simulink model "PID"  (R2017a)
settings: Solver=ode45  StartTime=0.0  StopTime=10.0  RelTol=1e-3  EnableMultiTasking=on
libraries: powerlib_meascontrol x3, simulink x1
settings Model: Creator=fangtiqiang  LastModifiedBy=fangtiqiang
settings DataIOCC: LimitDataPoints=on  SaveFormat=Array
settings OptimizationCC: LifeSpan=inf
settings DebuggingCC: SolverPrmCheckMsg=warning  SFUnexpectedBacktrackingDiag=warning  SFNoUnconditionalDefaultTransitionDiag=warning  SFExecutionAtInitializationDiag=none
settings HardwareCC: ProdBitPerPointer=32  ProdBitPerSizeT=32  ProdBitPerPtrDiffT=32  ProdLargestAtomicFloat=None  ProdIntDivRoundTo=Undefined  ProdEndianess=Unspecified  ProdWordSize=32  ProdHWDeviceType=32-bit Generic
settings ModelReferenceCC: PropagateSignalLabelsOutOfModel=off
settings GRTTargetCC: TargetLangStandard=C89/C90 (ANSI)  GeneratePreprocessorConditionals=Disable all
settings ConfigComp: CovMetricSettings=dw  CovHtmlReporting=on  CovSaveCumulativeToWorkspaceVar=on  CovSaveSingleToWorkspaceVar=on  CovExternalEMLEnable=off  CovSFcnEnable=off

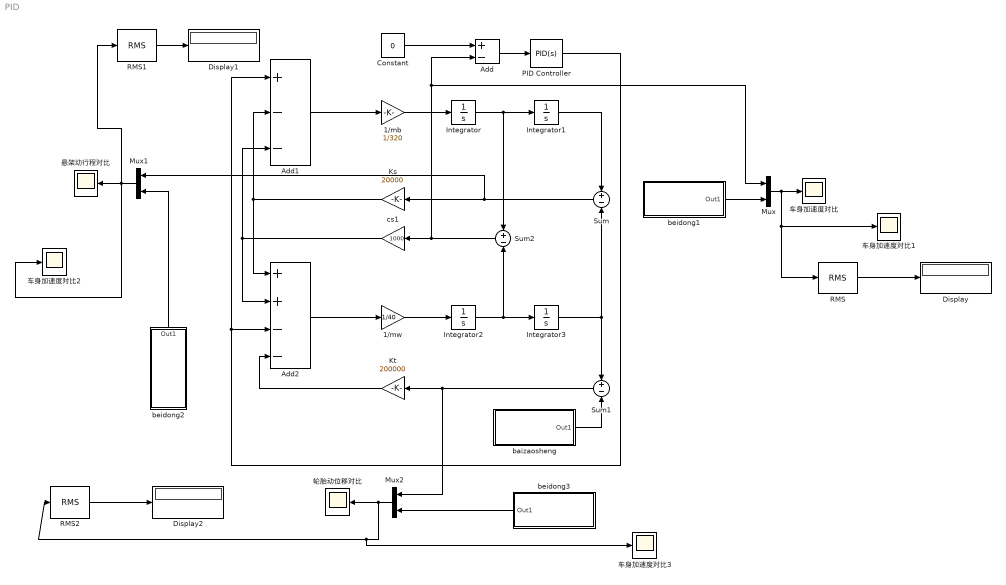
== system PID ==
  1/mb : Gain  Gain=1/320
  1/mw : Gain  Gain=1/40
  Add : Sum  Inputs=+-
  Add1 : Sum  Inputs=+--
  Add2 : Sum  Inputs=++--
  Constant : Constant  Value=0
  Display : Display
  Display1 : Display
  Display2 : Display
  Integrator{,1..3} (4 alike) : Integrator
  Ks : Gain  Gain=20000
  Kt : Gain  Gain=200000
  Mux : Mux  Inputs=2
  Mux1 : Mux  Inputs=2
  Mux2 : Mux  Inputs=2
  PID Controller : simulink/Continuous/PID Controller  Controller=PID  TimeDomain=Continuous-time  SampleTime=-1  IntegratorMethod=Forward Euler  FilterMethod=Forward Euler  Form=Parallel  UseFilter=on  ControllerParametersSource=internal  P=500  I=10  D=1  N=100  InitialConditionSource=internal  InitialConditionForIntegrator=0  InitialConditionForFilter=0  ExternalReset=none  LimitOutput=off  UpperSaturationLimit=inf  LowerSaturationLimit=-inf  LinearizeAsGain=on  AntiWindupMode=none  Kb=1  TrackingMode=off  Kt=1  PParamMin=[]  PParamMax=[]  IParamMin=[]  IParamMax=[]  DParamMin=[]  DParamMax=[]  NParamMin=[]  NParamMax=[]  KbParamMin=[]  KbParamMax=[]  KtParamMin=[]  KtParamMax=[]  POutMin=[]  POutMax=[]  IOutMin=[]  IOutMax=[]  DOutMin=[]  DOutMax=[]  NOutMin=[]  NOutMax=[]  KbOutMin=[]  KbOutMax=[]  KtOutMin=[]  KtOutMax=[]  IntegratorOutMin=[]  IntegratorOutMax=[]  FilterOutMin=[]  FilterOutMax=[]  SumOutMin=[]  SumOutMax=[]  SumI1OutMin=[]  SumI1OutMax=[]  SumI2OutMin=[]  SumI2OutMax=[]  SumI3OutMin=[]  SumI3OutMax=[]  SumDOutMin=[]  SumDOutMax=[]  SaturationOutMin=[]  SaturationOutMax=[]  IntegratorContinuousStateAttributes=''  IntegratorStateMustResolveToSignalObject=off  IntegratorRTWStateStorageClass=Auto  FilterContinuousStateAttributes=''  FilterStateMustResolveToSignalObject=off  FilterRTWStateStorageClass=Auto  DifferentiatorICPrevScaledInput=0  DifferentiatorOutMin=[]  DifferentiatorOutMax=[]  InitialConditionSetting=State (most efficient)
  RMS : powerlib_meascontrol/Measurements/RMS  TrueRMS=on  Freq=60  RMSInit=120  Ts=0
  RMS1 : powerlib_meascontrol/Measurements/RMS  TrueRMS=on  Freq=60  RMSInit=120  Ts=0
  RMS2 : powerlib_meascontrol/Measurements/RMS  TrueRMS=on  Freq=60  RMSInit=120  Ts=0
  Sum : Sum  Inputs=+-
  Sum1 : Sum  Inputs=+-
  Sum2 : Sum  Inputs=+-
  baizaosheng : Subsystem
  beidong1 : Subsystem
  beidong2 : Subsystem
  beidong3 : Subsystem
  cs1 : Gain  Gain=1000
  悬架动行程对比 : Scope
  车身加速度对比{,1..3} (4 alike) : Scope
  轮胎动位移对比 : Scope
  wires:
  1/mb/1 -> Integrator/1
  Integrator/1 -> Sum2/1, Integrator1/1
  Integrator1/1 -> Sum/1
  Sum/1 -> Mux1/1, Ks/1
  Integrator3/1 -> Sum/2, Sum1/1
  1/mw/1 -> Integrator2/1
  Integrator2/1 -> Sum2/2, Integrator3/1
  Sum1/1 -> Mux2/1, Kt/1
  Ks/1 -> Add1/2, Add2/1
  baizaosheng/1(Out1) -> Sum1/2
  Add1/1 -> 1/mb/1
  Add2/1 -> 1/mw/1
  Sum2/1 -> Add/2, Mux/1, cs1/1
  Kt/1 -> Add2/4
  cs1/1 -> Add2/2, Add1/3
  Add/1 -> PID Controller/1
  Constant/1 -> Add/1
  PID Controller/1 -> Add2/3, Add1/1
  Mux/1 -> 车身加速度对比/1, 车身加速度对比1/1, RMS/1
  beidong1/1(Out1) -> Mux/2
  RMS/1 -> Display/1
  RMS1/1 -> Display1/1
  beidong2/1(Out1) -> Mux1/2
  Mux1/1 -> 车身加速度对比2/1, RMS1/1, 悬架动行程对比/1
  beidong3/1(Out1) -> Mux2/2
  Mux2/1 -> 车身加速度对比3/1, RMS2/1, 轮胎动位移对比/1
  RMS2/1 -> Display2/1

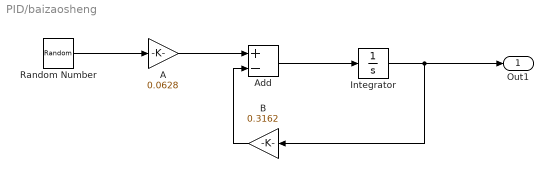
== system PID/baizaosheng ==
  A : Gain  Gain=0.0628
  Add : Sum  Inputs=+-
  B : Gain  Gain=0.3162
  Integrator : Integrator
  Random Number : RandomNumber  SampleTime=0.1
  Out1 : Outport
  wires:
  Random Number/1 -> A/1
  A/1 -> Add/1
  Add/1 -> Integrator/1
  Integrator/1 -> Out1/1, B/1
  B/1 -> Add/2

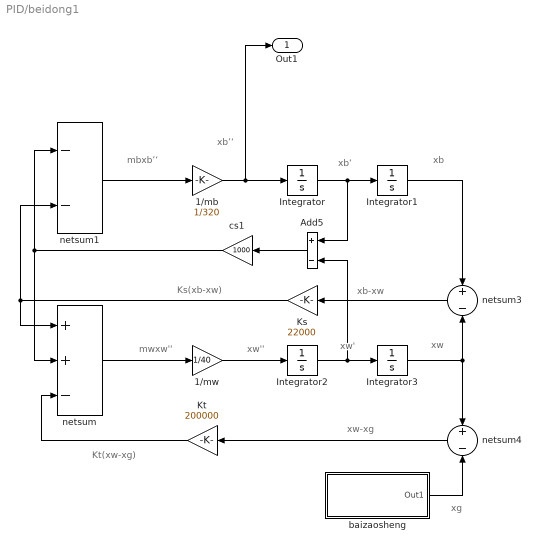
== system PID/beidong1 ==
  note: mwxw''
  note: xw''
  note: xw'
  note: mbxb’‘
  note: xb’‘
  note: xb‘
  note: Kt(xw-xg)
  note: xw-xg
  note: xg
  note: Ks(xb-xw)
  note: xb-xw
  note: xw
  note: xb
  1/mb : Gain  Gain=1/320
  1/mw : Gain  Gain=1/40
  Add5 : Sum  Inputs=+-
  Integrator{,1..3} (4 alike) : Integrator
  Ks : Gain  Gain=22000
  Kt : Gain  Gain=200000
  baizaosheng : Subsystem
  cs1 : Gain  Gain=1000
  netsum : Sum  Inputs=++-  SaturateOnIntegerOverflow=on  InputSameDT=on  OutDataTypeStr=Inherit: Same as first input
  netsum1 : Sum  Inputs=--  SaturateOnIntegerOverflow=on  InputSameDT=on  OutDataTypeStr=Inherit: Same as first input
  netsum3 : Sum  Inputs=+-  SaturateOnIntegerOverflow=on  InputSameDT=on  OutDataTypeStr=Inherit: Same as first input
  netsum4 : Sum  Inputs=+-  SaturateOnIntegerOverflow=on  InputSameDT=on  OutDataTypeStr=Inherit: Same as first input
  Out1 : Outport
  wires:
  netsum1/1 -> 1/mb/1
  1/mb/1 -> Out1/1, Integrator/1
  Integrator/1 -> Add5/1, Integrator1/1
  Integrator1/1 -> netsum3/1
  netsum3/1 -> Ks/1
  Integrator3/1 -> netsum4/1, netsum3/2
  netsum/1 -> 1/mw/1
  1/mw/1 -> Integrator2/1
  Integrator2/1 -> Integrator3/1, Add5/2
  netsum4/1 -> Kt/1
  Ks/1 -> netsum1/2, netsum/1
  Kt/1 -> netsum/3
  baizaosheng/1(Out1) -> netsum4/2
  Add5/1 -> cs1/1
  cs1/1 -> netsum1/1, netsum/2

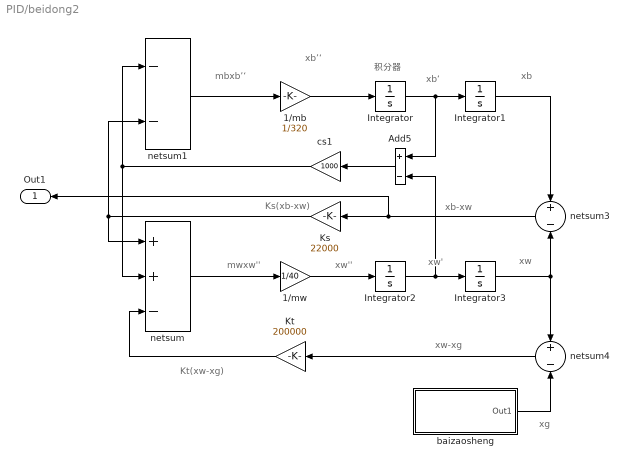
== system PID/beidong2 ==
  note: mwxw''
  note: xw''
  note: xw'
  note: mbxb’‘
  note: xb’‘
  note: xb‘
  note: 积分器
  note: Kt(xw-xg)
  note: xw-xg
  note: xg
  note: Ks(xb-xw)
  note: xb-xw
  note: xw
  note: xb
  1/mb : Gain  Gain=1/320
  1/mw : Gain  Gain=1/40
  Add5 : Sum  Inputs=+-
  Integrator{,1..3} (4 alike) : Integrator
  Ks : Gain  Gain=22000
  Kt : Gain  Gain=200000
  baizaosheng : Subsystem
  cs1 : Gain  Gain=1000
  netsum : Sum  Inputs=++-  SaturateOnIntegerOverflow=on  InputSameDT=on  OutDataTypeStr=Inherit: Same as first input
  netsum1 : Sum  Inputs=--  SaturateOnIntegerOverflow=on  InputSameDT=on  OutDataTypeStr=Inherit: Same as first input
  netsum3 : Sum  Inputs=+-  SaturateOnIntegerOverflow=on  InputSameDT=on  OutDataTypeStr=Inherit: Same as first input
  netsum4 : Sum  Inputs=+-  SaturateOnIntegerOverflow=on  InputSameDT=on  OutDataTypeStr=Inherit: Same as first input
  Out1 : Outport
  wires:
  netsum1/1 -> 1/mb/1
  1/mb/1 -> Integrator/1
  Integrator/1 -> Add5/1, Integrator1/1
  Integrator1/1 -> netsum3/1
  netsum3/1 -> Out1/1, Ks/1
  Integrator3/1 -> netsum4/1, netsum3/2
  netsum/1 -> 1/mw/1
  1/mw/1 -> Integrator2/1
  Integrator2/1 -> Integrator3/1, Add5/2
  netsum4/1 -> Kt/1
  Ks/1 -> netsum1/2, netsum/1
  Kt/1 -> netsum/3
  baizaosheng/1(Out1) -> netsum4/2
  cs1/1 -> netsum1/1, netsum/2
  Add5/1 -> cs1/1

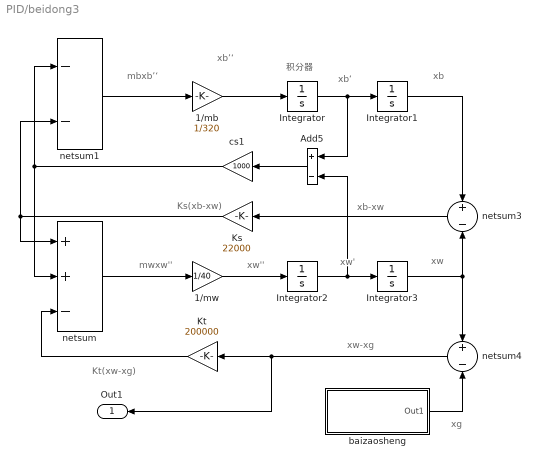
== system PID/beidong3 ==
  note: mwxw''
  note: xw''
  note: xw'
  note: mbxb’‘
  note: xb’‘
  note: xb‘
  note: 积分器
  note: Kt(xw-xg)
  note: xw-xg
  note: xg
  note: Ks(xb-xw)
  note: xb-xw
  note: xw
  note: xb
  1/mb : Gain  Gain=1/320
  1/mw : Gain  Gain=1/40
  Add5 : Sum  Inputs=+-
  Integrator{,1..3} (4 alike) : Integrator
  Ks : Gain  Gain=22000
  Kt : Gain  Gain=200000
  baizaosheng : Subsystem
  cs1 : Gain  Gain=1000
  netsum : Sum  Inputs=++-  SaturateOnIntegerOverflow=on  InputSameDT=on  OutDataTypeStr=Inherit: Same as first input
  netsum1 : Sum  Inputs=--  SaturateOnIntegerOverflow=on  InputSameDT=on  OutDataTypeStr=Inherit: Same as first input
  netsum3 : Sum  Inputs=+-  SaturateOnIntegerOverflow=on  InputSameDT=on  OutDataTypeStr=Inherit: Same as first input
  netsum4 : Sum  Inputs=+-  SaturateOnIntegerOverflow=on  InputSameDT=on  OutDataTypeStr=Inherit: Same as first input
  Out1 : Outport
  wires:
  netsum1/1 -> 1/mb/1
  1/mb/1 -> Integrator/1
  Integrator/1 -> Add5/1, Integrator1/1
  Integrator1/1 -> netsum3/1
  netsum3/1 -> Ks/1
  Integrator3/1 -> netsum4/1, netsum3/2
  netsum/1 -> 1/mw/1
  1/mw/1 -> Integrator2/1
  Integrator2/1 -> Integrator3/1, Add5/2
  netsum4/1 -> Out1/1, Kt/1
  Ks/1 -> netsum1/2, netsum/1
  Kt/1 -> netsum/3
  baizaosheng/1(Out1) -> netsum4/2
  Add5/1 -> cs1/1
  cs1/1 -> netsum1/1, netsum/2

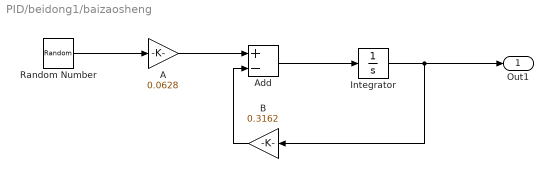
== system PID/beidong1/baizaosheng ==
  A : Gain  Gain=0.0628
  Add : Sum  Inputs=+-
  B : Gain  Gain=0.3162
  Integrator : Integrator
  Random Number : RandomNumber  SampleTime=0.1
  Out1 : Outport
  wires:
  Random Number/1 -> A/1
  A/1 -> Add/1
  Add/1 -> Integrator/1
  Integrator/1 -> Out1/1, B/1
  B/1 -> Add/2

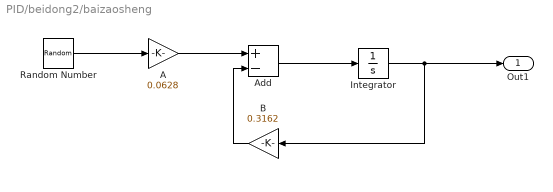
== system PID/beidong2/baizaosheng ==
  A : Gain  Gain=0.0628
  Add : Sum  Inputs=+-
  B : Gain  Gain=0.3162
  Integrator : Integrator
  Random Number : RandomNumber  SampleTime=0.1
  Out1 : Outport
  wires:
  Random Number/1 -> A/1
  A/1 -> Add/1
  Add/1 -> Integrator/1
  Integrator/1 -> Out1/1, B/1
  B/1 -> Add/2

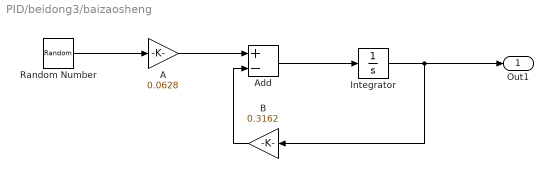
== system PID/beidong3/baizaosheng ==
  A : Gain  Gain=0.0628
  Add : Sum  Inputs=+-
  B : Gain  Gain=0.3162
  Integrator : Integrator
  Random Number : RandomNumber  SampleTime=0.1
  Out1 : Outport
  wires:
  Random Number/1 -> A/1
  A/1 -> Add/1
  Add/1 -> Integrator/1
  Integrator/1 -> Out1/1, B/1
  B/1 -> Add/2
